simulink model "cascaderegulering"  (Simulink 7.4)
settings: Solver=ode4  StartTime=0.0  StopTime=inf  FixedStep=0.01  RelTol=1e-3
values from neighbouring files (symbols this model uses):
  aarm = -15.836    [cascadereguleringStart.m]    (also in testsensorStart.m)
  apind = -16.85    [cascadereguleringStart.m]    (also in testsensorStart.m)
  bpind = -0.0674    [cascadereguleringStart.m]    (also in testsensorStart.m = 0.6)
undefined symbols (not defined in the file or in its folder): kd, kff, ki, Ti
libraries: xpcnilib x2
settings Model: Creator=Skov  LastModifiedBy=Skov  SimulationMode=external  BufferReuse=off
settings DataIOCC: SaveState=on  InspectSignalLogs=on
settings OptimizationCC: BlockReduction=off  OptimizeBlockIOStorage=off  BufferReuse=off  ExpressionFolding=off  LocalBlockOutputs=off
settings HardwareCC: ProdIntDivRoundTo=Zero  ProdEndianess=LittleEndian  ProdHWDeviceType=Generic->32-bit x86 compatible
settings RTWCC: SystemTargetFile=xpctarget.tlc  TemplateMakefile=xpc_default_tmf  Description=xPC Target  ProcessScript=xpctarget_make_rtw_hook  RTWCompilerOptimization=On
settings xpcTargetCC: TargetFcnLib=ansi_tfl_table_tmw.mat  TargetFunctionLibrary=ANSI_C  ParMdlRefBuildCompliant=off  PortableWordSizes=off  xPCLoadParamSetFile=off

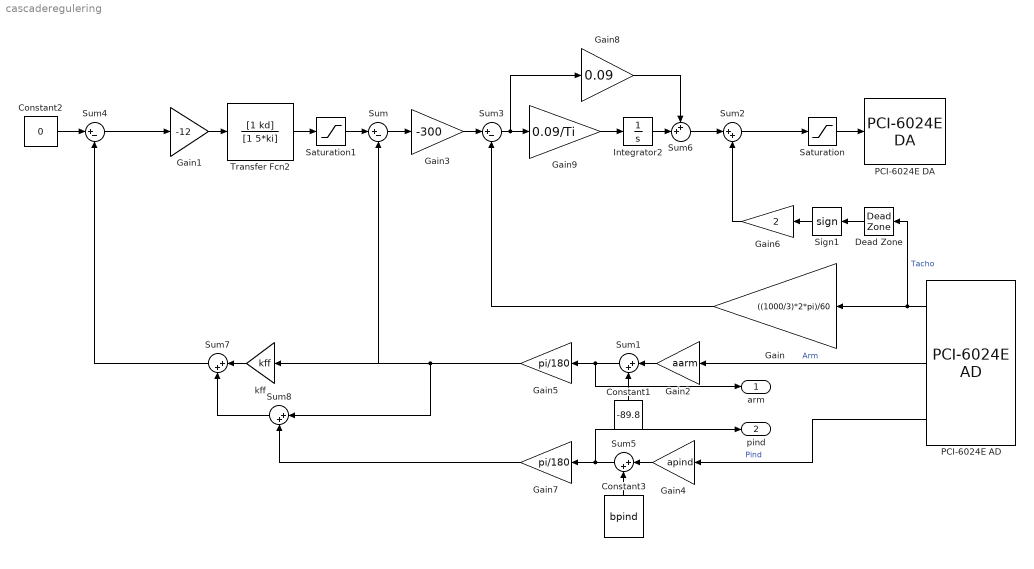
== system cascaderegulering ==
  Constant1 : Constant  Value=-89.8  OutDataType=fixdt(1, 16)  OutScaling=2^0
  Constant2 : Constant  Value=0  OutDataType=fixdt(1, 16)  OutScaling=2^0
  Constant3 : Constant  Value=bpind  OutDataType=fixdt(1, 16)  OutScaling=2^0
  Dead Zone : DeadZone  LowerValue=-0.1  UpperValue=0.1  SaturateOnIntegerOverflow=on
  Gain : Gain  Gain=((1000/3)*2*pi)/60  ParameterDataType=fixdt(1, 16)  ParameterScaling=2^0  OutDataType=fixdt(1, 16)  OutScaling=2^0
  Gain1 : Gain  Gain=-12  ParameterDataType=fixdt(1, 16)  ParameterScaling=2^0  OutDataType=fixdt(1, 16)  OutScaling=2^0
  Gain2 : Gain  Gain=aarm  ParameterDataType=fixdt(1, 16)  ParameterScaling=2^0  OutDataType=fixdt(1, 16)  OutScaling=2^0
  Gain3 : Gain  Gain=-300  ParameterDataType=fixdt(1, 16)  ParameterScaling=2^0  OutDataType=fixdt(1, 16)  OutScaling=2^0
  Gain4 : Gain  Gain=apind  ParameterDataType=fixdt(1, 16)  ParameterScaling=2^0  OutDataType=fixdt(1, 16)  OutScaling=2^0
  Gain5 : Gain  Gain=pi/180  ParameterDataType=fixdt(1, 16)  ParameterScaling=2^0  OutDataType=fixdt(1, 16)  OutScaling=2^0
  Gain6 : Gain  Gain=2  ParameterDataType=fixdt(1, 16)  ParameterScaling=2^0  OutDataType=fixdt(1, 16)  OutScaling=2^0
  Gain7 : Gain  Gain=pi/180  ParameterDataType=fixdt(1, 16)  ParameterScaling=2^0  OutDataType=fixdt(1, 16)  OutScaling=2^0
  Gain8 : Gain  Gain=0.09  ParameterDataType=fixdt(1, 16)  ParameterScaling=2^0  OutDataType=fixdt(1, 16)  OutScaling=2^0
  Gain9 : Gain  Gain=0.09/Ti  ParameterDataType=fixdt(1, 16)  ParameterScaling=2^0  OutDataType=fixdt(1, 16)  OutScaling=2^0
  Integrator2 : Integrator
  PCI-6024E AD : xpcnilib/A//D/E Series/PCI-6024E AD  channel=[3 1 2]  range=[-10]  coupling=[0]  sampletime=0.01  slot=-1
  PCI-6024E DA : xpcnilib/D//A/E Series/PCI-6024E DA  channel=[1]  reset=[1]  initValue=[0]  sampletime=0.01  slot=-1
  Saturation : Saturate  UpperLimit=10  LowerLimit=-10  OutDataType=fixdt(1, 16)  OutScaling=2^0
  Saturation1 : Saturate  UpperLimit=pi/3  LowerLimit=-pi/3  OutDataType=fixdt(1, 16)  OutScaling=2^0
  Sign1 : Signum
  Sum : Sum  Inputs=|+-  OutDataType=fixdt(1, 16)  OutScaling=2^0
  Sum{1..2,5,7..8} (5 alike) : Sum  Inputs=|++  OutDataType=fixdt(1, 16)  OutScaling=2^0
  Sum3 : Sum  Inputs=|+-  OutDataType=fixdt(1, 16)  OutScaling=2^0
  Sum4 : Sum  Inputs=|+-  OutDataType=fixdt(1, 16)  OutScaling=2^0
  Sum6 : Sum  Inputs=++|  OutDataType=fixdt(1, 16)  OutScaling=2^0
  Transfer Fcn2 : TransferFcn  Numerator=[1 kd]  Denominator=[1 5*ki]
  kff : Gain  Gain=kff  ParameterDataType=fixdt(1, 16)  ParameterScaling=2^0  OutDataType=fixdt(1, 16)  OutScaling=2^0
  arm : Outport  OutDataType=fixdt(1, 16)  OutScaling=2^0
  pind : Outport  Port=2  OutDataType=fixdt(1, 16)  OutScaling=2^0
  wires:
  Sum/1 -> Gain3/1
  Gain/1 -> Sum3/2
  Gain2/1 -> Sum1/1
  Constant1/1 -> Sum1/2
  Gain3/1 -> Sum3/1
  Sum1/1 -> Gain5/1, arm/1
  PCI-6024E AD/1 -> Gain/1, Dead Zone/1  "Tacho"
  PCI-6024E AD/2 -> Gain2/1  "Arm"
  Gain5/1 -> kff/1, Sum/2, Sum8/1
  Sum2/1 -> Saturation/1
  PCI-6024E AD/3 -> Gain4/1  "Pind"
  Constant2/1 -> Sum4/1
  Gain4/1 -> Sum5/1
  Constant3/1 -> Sum5/2
  Sum5/1 -> Gain7/1, pind/1
  Saturation/1 -> PCI-6024E DA/1
  Dead Zone/1 -> Sign1/1
  Sign1/1 -> Gain6/1
  Gain6/1 -> Sum2/2
  Gain1/1 -> Transfer Fcn2/1
  Sum4/1 -> Gain1/1
  Gain9/1 -> Integrator2/1
  Integrator2/1 -> Sum6/2
  Gain8/1 -> Sum6/1
  Sum3/1 -> Gain8/1, Gain9/1
  Sum6/1 -> Sum2/1
  kff/1 -> Sum7/1
  Sum7/1 -> Sum4/2
  Gain7/1 -> Sum8/2
  Sum8/1 -> Sum7/2
  Transfer Fcn2/1 -> Saturation1/1
  Saturation1/1 -> Sum/1
